simulink model "MG_2018b"  (R2020a)
settings: Solver=ode1  StartTime=0.0  StopTime=inf  FixedStep=2e-5  RelTol=1e-3  EnableMultiTasking=on
libraries: powerlib x26, powerlib_meascontrol x5, rtlab x3
settings Model: ARTEMISmethode_block_infos=$$__separator__$$  Creator=pengf  LastModifiedBy=mzh
settings SolverCC: AutoInsertRateTranBlk=on
settings DataIOCC: LimitDataPoints=on  SaveFormat=Array  SaveOutput=off  SaveTime=off  ReturnWorkspaceOutputs=off
settings OptimizationCC: LocalBlockOutputs=off  LifeSpan=inf
settings DebuggingCC: UnderspecifiedInitializationDetection=Classic  CheckExecutionContextPreStartOutputMsg=on  CheckExecutionContextRuntimeOutputMsg=on  SFUnexpectedBacktrackingDiag=warning  SFNoUnconditionalDefaultTransitionDiag=warning  SFExecutionAtInitializationDiag=none  ArithmeticOperatorsInVariantConditions=warning
settings HardwareCC: ProdBitPerPointer=32  ProdBitPerSizeT=32  ProdBitPerPtrDiffT=32  ProdLargestAtomicFloat=None  ProdIntDivRoundTo=Undefined  ProdEndianess=Unspecified  ProdWordSize=32  ProdHWDeviceType=32-bit Generic
settings ModelReferenceCC: PropagateSignalLabelsOutOfModel=off
settings SFSimCC: SimUseLocalCustomCode=off  CustomCodeUndefinedFunction=UseInterfaceOnly
settings RTWCC: RTWUseLocalCustomCode=off
settings CodeAppCC: StateflowObjectComments=on
settings GRTTargetCC: TargetLangStandard=C89/C90 (ANSI)  CombineOutputUpdateFcns=off  GRTInterface=on
settings ConfigComp: CovMetricSettings=dw  CovHtmlReporting=on  CovSaveCumulativeToWorkspaceVar=on  CovSaveSingleToWorkspaceVar=on  CovExternalEMLEnable=off
settings SimscapeCC: SimscapeNormalizeSystem=off

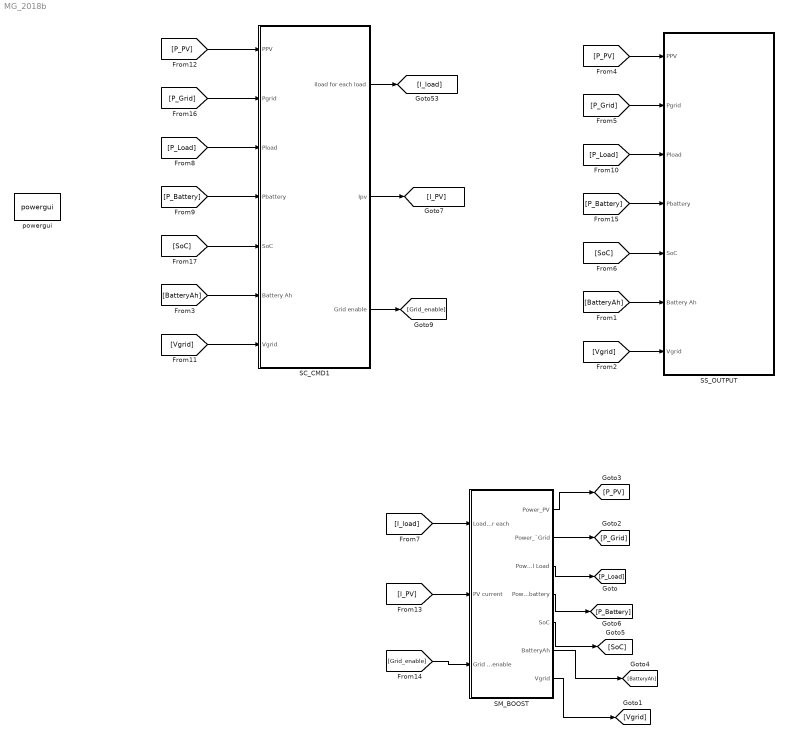
== system MG_2018b ==
  SC_CMD1 : Subsystem
  SM_BOOST : Subsystem
  SS_OUTPUT : Subsystem
  powergui : powerlib/powergui  Priority=1  SimulationMode=Discrete  SampleTime=2e-5  frequency=60  Iterations=50  frequencyindice=60  Pbase=100e6  ErrMax=1e-4  UnitsV=kV  UnitsW=MW  buscounter=0  FunctionMessages=off  echomessages=off  EnableUseOfTLC=off  CurrentSourceSwitches=off  DisableSnubberDevices=off  DisableRonSwitches=off  DisableVfSwitches=off  DisplayEquations=off  AutomaticDiscreteSolvers=off  SolverType=Tustin  Interpol=off  ExternalGateDelay=off  methode=off  Ts=100  x0status=blocks  SPID=off  SwTol=0  HookPort=off  NonlinearTolerance=1e-4  nMaxIteration=100  ContinueOnMaxIteration=off  RestoreLinks=warning  ResistiveCurrentMeasurement=off  Frange=[0:2:500]  Ylog=off  Xlog=on  ShowGrid=off  save=off  variable=ZData  structure=ScopeData3  ZoomFFT=off  StartTime=0.1  cycles=2  DisplayStyle=3  fundamental=50  FreqAxis=off  MaxFrequency=1000  frequencyindicesteady=1  RmsSteady=1  display=off
  wires:
  SC_CMD1/1(Iload for each load) -> [I_load]
  [P_PV] -> SC_CMD1/1(PPV)
  [P_Grid] -> SC_CMD1/2(Pgrid)
  [P_Grid] -> SS_OUTPUT/2(Pgrid)
  [I_load] -> SM_BOOST/1(Load current for each)
  [P_Battery] -> SC_CMD1/4(Pbattery)
  [SoC] -> SC_CMD1/5(SoC)
  [P_Battery] -> SS_OUTPUT/4(Pbattery)
  [Vgrid] -> SC_CMD1/7(Vgrid)
  [SoC] -> SS_OUTPUT/5(SoC)
  [P_Load] -> SC_CMD1/3("Pload ")
  [BatteryAh] -> SC_CMD1/6(Battery Ah)
  [P_PV] -> SS_OUTPUT/1(PPV)
  [P_Load] -> SS_OUTPUT/3("Pload ")
  SC_CMD1/2(Ipv) -> [I_PV]
  [I_PV] -> SM_BOOST/2(PV current)
  SM_BOOST/1(Power_PV) -> [P_PV]
  SM_BOOST/2(Power_`Grid) -> [P_Grid]
  SM_BOOST/3(Power_Total Load) -> [P_Load]
  SM_BOOST/4(Power_battery) -> [P_Battery]
  SM_BOOST/5(SoC) -> [SoC]
  SM_BOOST/6(BatteryAh) -> [BatteryAh]
  [Grid_enable] -> SM_BOOST/3(Grid connection enable)
  SM_BOOST/7("Vgrid ") -> [Vgrid]
  [BatteryAh] -> SS_OUTPUT/6(Battery Ah)
  [Vgrid] -> SS_OUTPUT/7(Vgrid)
  SC_CMD1/3(Grid enable) -> [Grid_enable]

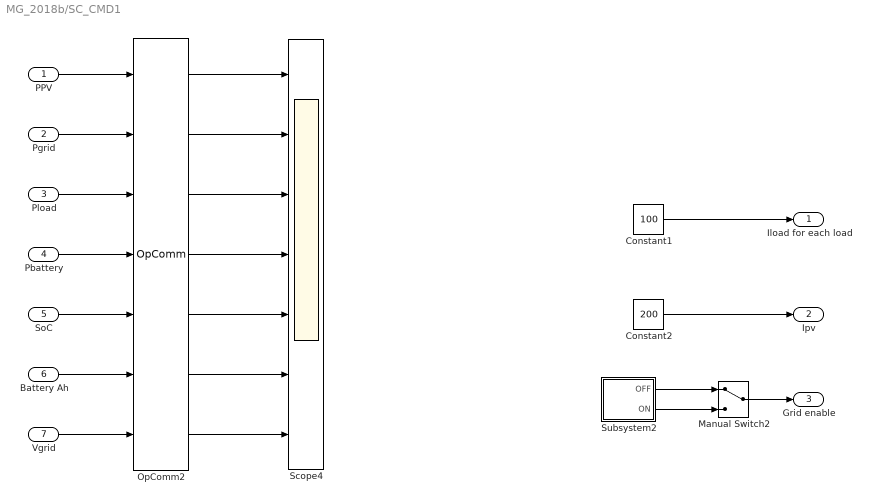
== system MG_2018b/SC_CMD1 ==
  PPV : Inport
  Pgrid : Inport  Port=2
  "Pload " : Inport  Port=3
  Pbattery : Inport  Port=4
  SoC : Inport  Port=5
  Battery Ah : Inport  Port=6
  Vgrid : Inport  Port=7
  Constant1 : Constant  Value=100
  Constant2 : Constant  Value=200
  Manual Switch2 : ManualSwitch
  OpComm2 : rtlab/OpComm  nbport=7  groupe_acq=1  subsys_rate=0  st=0  Synchronization=on  Interpolation=on  Threshold=1.0  Missed_Data=off  Sim_Time=off  Samples=off  dynSigOut=off  from_console=0  warning_done=off  writeOpCommFile=off  Offset=off
      settings: SourceProductName=RT-LAB
  Scope4 : Scope  NumInputPorts=7
  Subsystem2 : Subsystem
  Iload for each load : Outport
  Ipv : Outport  Port=2
  Grid enable : Outport  Port=3
  wires:
  Constant1/1 -> Iload for each load/1
  PPV/1 -> OpComm2/1
  Pgrid/1 -> OpComm2/2
  Pbattery/1 -> OpComm2/4
  SoC/1 -> OpComm2/5
  "Pload "/1 -> OpComm2/3
  Battery Ah/1 -> OpComm2/6
  Vgrid/1 -> OpComm2/7
  Constant2/1 -> Ipv/1
  OpComm2/1 -> Scope4/1
  OpComm2/2 -> Scope4/2
  OpComm2/3 -> Scope4/3
  OpComm2/4 -> Scope4/4
  OpComm2/5 -> Scope4/5
  OpComm2/6 -> Scope4/6
  OpComm2/7 -> Scope4/7
  Subsystem2/1(OFF) -> Manual Switch2/1
  Subsystem2/2(ON) -> Manual Switch2/2
  Manual Switch2/1 -> Grid enable/1

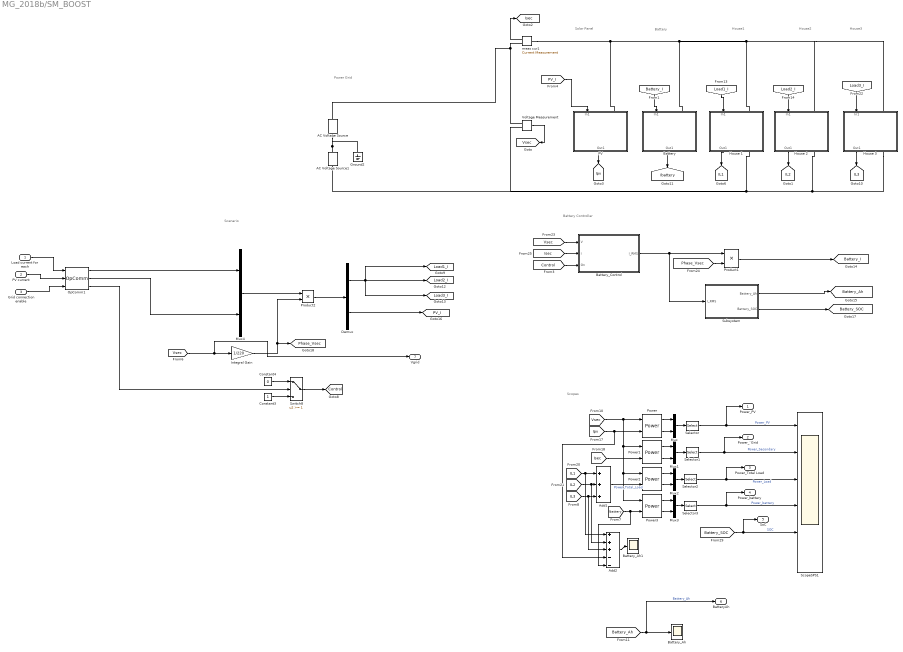
== system MG_2018b/SM_BOOST ==
  note: House1
  note: Solar Panel
  note: Scopes
  note: House3
  note: Battery Controller
  note: Battery
  note: House2
  note: Power Grid
  note: Scenario
  Load current for each : Inport
  PV current : Inport  Port=2
  Grid connection enable : Inport  Port=3
  AC Voltage Source : powerlib/Electrical Sources/AC Voltage Source  Amplitude=110  Phase=0  Frequency=60  SampleTime=0  Measurements=None  BusType=swing  Pref=10e3  Qref=0  Qmin=-inf  Qmax=+inf
  AC Voltage Source1 : powerlib/Electrical Sources/AC Voltage Source  Amplitude=110  Phase=0  Frequency=60  SampleTime=0  Measurements=None  BusType=swing  Pref=10e3  Qref=0  Qmin=-inf  Qmax=+inf
  Add1 : Sum  Inputs=+++
  Add2 : Sum  Inputs=+++--
  Battery : Subsystem
  Battery_Ah : Scope
  Battery_Ah1 : Scope
  Battery_Control : Subsystem
  Constant3 : Constant
  Constant4 : Constant  Value=0
  Demux : Demux  Outputs=2
  Ground2 : powerlib/Elements/Ground  LConnTagsString=a
  House 1 : Subsystem
  House 2 : Subsystem
  House 3 : Subsystem
  Integral Gain : Gain  Gain=1/220
  Mux{,1..4} (5 alike) : Mux  Inputs=2
  OpComm1 : rtlab/OpComm  nbport=3  groupe_acq=1  subsys_rate=0  st=0  Synchronization=on  Interpolation=on  Threshold=1.0  Missed_Data=off  Sim_Time=off  Samples=off  dynSigOut=off  from_console=1  warning_done=off  writeOpCommFile=off  Offset=off
      settings: SourceProductName=RT-LAB
  PV : Subsystem
  Power{,1..3} (4 alike) : powerlib_meascontrol/Measurements/Power  Freq=60  Vinit=[1, 0]  Iinit=[1, 0]  Ts=0
  Product1 : Product
  Product2 : Product
  ScopeSPS1 : Scope  NumInputPorts=6
  Selector{,1..3} (4 alike) : Selector  InputPortWidth=2  IndexOptions=Index vector (dialog)  Indices=1  OutputSizes=1
  Subsystem : Subsystem  mask{AH=100}
      mask prompts: AH "Capacity[Ah]"
  Switch8 : Switch  Threshold=1
  Voltage Measurement : powerlib/Measurements/Voltage Measurement  PhasorSimulation=off  OutputType=Complex  PSBequivalent=0
  meas cur1 : powerlib/Measurements/Current Measurement  PhasorSimulation=off  OutputType=Complex  PSBequivalent=0
  Power_PV : Outport
  Power_`Grid : Outport  Port=2
  Power_Total Load : Outport  Port=3
  Power_battery : Outport  Port=4
  SoC : Outport  Port=5
  BatteryAh : Outport  Port=6
  "Vgrid " : Outport  Port=7
  tag scope: Battery_Ah=global, Battery_I=global, Battery_SOC=global, Control=global, IL1=global, IL2=global, IL3=global, Ibattery=global, Ipv=global, Isec=global, Load1_I=global, Load2_I=global, Load3_I=global, PV_I=global, Phase_Vsec=global, Vsec=global
  wires:
  Load current for each/1 -> OpComm1/1
  PV current/1 -> OpComm1/2
  [Load3_I] -> House 3/1(In1)
  House 1/1(Out1) -> [IL1]
  [Vsec] -> Battery_Control/1(V)
  [Load1_I] -> House 1/1(In1)
  [PV_I] -> PV/1(In1)
  Subsystem/1(Battery_Ah) -> [Battery_Ah]
  Battery/1(Out1) -> [Ibattery]
  [Battery_I] -> Battery/1(In1)
  Subsystem/2(Battery_SOC) -> [Battery_SOC]
  meas cur1/1 -> [Isec]
  [Control] -> Battery_Control/3(On)
  Battery_Control/1(I_RMS) -> Subsystem/1(I_RMS), Product1/1
  PV/1(Out1) -> [Ipv]
  House 2/1(Out1) -> [IL2]
  House 3/1(Out1) -> [IL3]
  [Isec] -> Battery_Control/2(I)
  [Phase_Vsec] -> Product1/2
  [Load2_I] -> House 2/1(In1)
  Voltage Measurement/1 -> [Vsec]
  Selector/1 -> Power_PV/1, ScopeSPS1/1  "Power_PV"
  [Vsec] -> Power1/1, Power3/1, Power2/1, Power/1
  Add1/1 -> Power2/2  "Power_Total_Load"
  [Isec] -> Power1/2
  [Ipv] -> Add2/4, Power/2
  Selector3/1 -> Power_battery/1, ScopeSPS1/4  "Power_battery"
  [Battery_SOC] -> SoC/1, ScopeSPS1/5  "SOC"
  [IL3] -> Add2/3, Add1/3
  Power/1 -> Mux/1
  [IL1] -> Add2/1, Add1/1
  [Battery_Ah] -> BatteryAh/1, Battery_Ah/1  "Battery_Ah"
  Power/2 -> Mux/2
  Selector2/1 -> Power_Total Load/1, ScopeSPS1/3  "Power_Load"
  Power1/1 -> Mux1/1
  Power3/2 -> Mux3/2
  Power2/1 -> Mux2/1
  Selector1/1 -> Power_`Grid/1, ScopeSPS1/2  "Power_Secondary"
  Power1/2 -> Mux1/2
  Power3/1 -> Mux3/1
  Mux3/1 -> Selector3/1
  Mux2/1 -> Selector2/1
  Mux/1 -> Selector/1
  Mux1/1 -> Selector1/1
  Add2/1 -> Battery_Ah1/1
  Power2/2 -> Mux2/2
  [Ibattery] -> Add2/5, Power3/2
  [IL2] -> Add2/2, Add1/2
  Mux4/1 -> Product2/1
  Integral Gain/1 -> [Phase_Vsec], Product2/2
  OpComm1/3 -> Switch8/2
  OpComm1/2 -> Mux4/2
  OpComm1/1 -> Mux4/1
  [Vsec] -> "Vgrid "/1, Integral Gain/1
  Constant3/1 -> Switch8/3
  Product2/1 -> Demux/1
  Constant4/1 -> Switch8/1
  Switch8/1 -> [Control]
  Grid connection enable/1 -> OpComm1/3
  Product1/1 -> [Battery_I]
  Demux/1 -> [Load3_I], [Load2_I], [Load1_I]
  Demux/2 -> [PV_I]
  connections:
  AC Voltage Source1/RConn1 -- AC Voltage Source/LConn1 -- Ground2/LConn1
  Voltage Measurement/LConn1 -- AC Voltage Source/RConn1 -- meas cur1/RConn1
  House 2/RConn1 -- House 3/RConn1 -- AC Voltage Source1/LConn1 -- Voltage Measurement/LConn2 -- House 1/RConn1
  Battery/LConn1 -- House 3/LConn1 -- House 2/LConn1 -- House 1/LConn1 -- meas cur1/LConn1 -- PV/LConn1

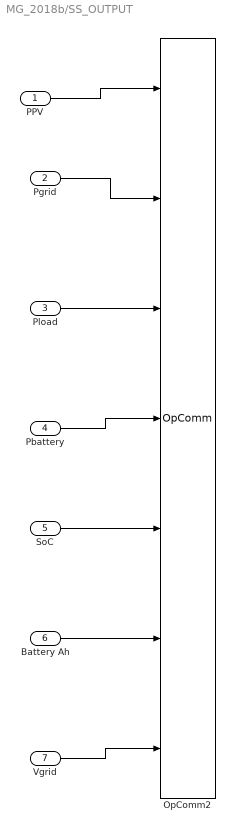
== system MG_2018b/SS_OUTPUT ==
  PPV : Inport
  Pgrid : Inport  Port=2
  "Pload " : Inport  Port=3
  Pbattery : Inport  Port=4
  SoC : Inport  Port=5
  Battery Ah : Inport  Port=6
  Vgrid : Inport  Port=7
  OpComm2 : rtlab/OpComm  nbport=7  groupe_acq=1  subsys_rate=0  st=0  Synchronization=on  Interpolation=on  Threshold=1.0  Missed_Data=off  Sim_Time=off  Samples=off  dynSigOut=off  from_console=0  warning_done=off  writeOpCommFile=off  Offset=off
      settings: SourceProductName=RT-LAB
  wires:
  Pgrid/1 -> OpComm2/2
  PPV/1 -> OpComm2/1
  "Pload "/1 -> OpComm2/3
  Pbattery/1 -> OpComm2/4
  SoC/1 -> OpComm2/5
  Battery Ah/1 -> OpComm2/6
  Vgrid/1 -> OpComm2/7

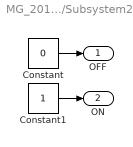
== system MG_2018b/SC_CMD1/Subsystem2 ==
  Constant : Constant  Value=0
  Constant1 : Constant
  OFF : Outport
  ON : Outport  Port=2
  wires:
  Constant/1 -> OFF/1
  Constant1/1 -> ON/1

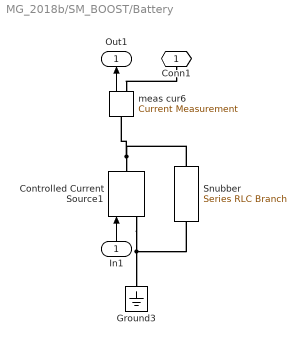
== system MG_2018b/SM_BOOST/Battery ==
  In1 : Inport
  Controlled Current Source1 : powerlib/Electrical Sources/Controlled Current Source  Initialize=on  Source_Type=AC  Amplitude=0  Phase=30  Frequency=60  Measurements=None
  Ground3 : powerlib/Elements/Ground  LConnTagsString=a
  Snubber : powerlib/Elements/Series RLC Branch  LConnTagsString=__new0  RConnTagsString=__new0  BranchType=R  Resistance=1e6  Inductance=1e-3  SetiL0=off  InitialCurrent=0  Capacitance=1e-6  Setx0=off  InitialVoltage=0  Measurements=None
  meas cur6 : powerlib/Measurements/Current Measurement  PhasorSimulation=off  OutputType=Complex  PSBequivalent=0
  Conn1 : PMIOPort  Side=Left
  Out1 : Outport  VectorParamsAs1DForOutWhenUnconnected=off
  wires:
  meas cur6/1 -> Out1/1
  In1/1 -> Controlled Current Source1/1
  connections:
  Controlled Current Source1/LConn1 -- Ground3/LConn1 -- Snubber/RConn1
  Controlled Current Source1/RConn1 -- Snubber/LConn1 -- meas cur6/LConn1
  Conn1/RConn1 -- meas cur6/RConn1

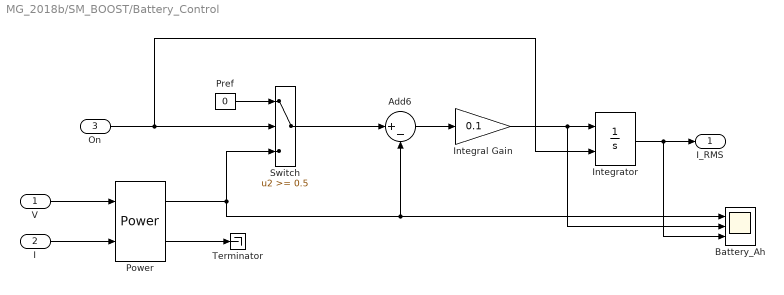
== system MG_2018b/SM_BOOST/Battery_Control ==
  V : Inport
  I : Inport  Port=2
  On : Inport  Port=3
  Add6 : Sum  Inputs=|+-
  Battery_Ah : Scope  NumInputPorts=3
  Integral Gain : Gain  Gain=0.1
  Integrator : Integrator  ExternalReset=falling  LimitOutput=on  UpperSaturationLimit=500  LowerSaturationLimit=-500
  Power : powerlib_meascontrol/Measurements/Power  Freq=60  Vinit=[1, 0]  Iinit=[1, 0]  Ts=0
  Pref : Constant  Value=0
  Switch : Switch  Threshold=0.5
  Terminator : Terminator
  I_RMS : Outport  OutputWhenDisabled=reset  InitialOutput=0  VectorParamsAs1DForOutWhenUnconnected=off
  wires:
  Pref/1 -> Switch/1
  Integrator/1 -> Battery_Ah/3, I_RMS/1
  On/1 -> Integrator/2, Switch/2
  Add6/1 -> Integral Gain/1
  Integral Gain/1 -> Battery_Ah/2, Integrator/1
  Power/1 -> Switch/3, Add6/2, Battery_Ah/1
  I/1 -> Power/2
  V/1 -> Power/1
  Power/2 -> Terminator/1
  Switch/1 -> Add6/1

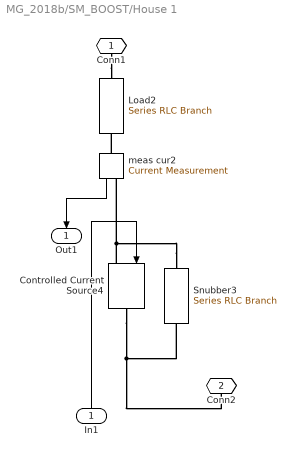
== system MG_2018b/SM_BOOST/House 1 ==
  In1 : Inport
  Controlled Current Source4 : powerlib/Electrical Sources/Controlled Current Source  Initialize=on  Source_Type=AC  Amplitude=0  Phase=30  Frequency=60  Measurements=None
  Load2 : powerlib/Elements/Series RLC Branch  LConnTagsString=__new0  RConnTagsString=__new0  BranchType=R  Resistance=16  Inductance=1e-3  SetiL0=off  InitialCurrent=0  Capacitance=1e-6  Setx0=off  InitialVoltage=0  Measurements=None
  Snubber3 : powerlib/Elements/Series RLC Branch  LConnTagsString=__new0  RConnTagsString=__new0  BranchType=R  Resistance=1e6  Inductance=1e-3  SetiL0=off  InitialCurrent=0  Capacitance=1e-6  Setx0=off  InitialVoltage=0  Measurements=None
  meas cur2 : powerlib/Measurements/Current Measurement  PhasorSimulation=off  OutputType=Complex  PSBequivalent=0
  Conn1 : PMIOPort  Side=Left
  Conn2 : PMIOPort  Port=2  Side=Right
  Out1 : Outport  VectorParamsAs1DForOutWhenUnconnected=off
  wires:
  In1/1 -> Controlled Current Source4/1
  meas cur2/1 -> Out1/1
  connections:
  Conn1/RConn1 -- Load2/LConn1
  meas cur2/LConn1 -- Load2/RConn1
  Snubber3/LConn1 -- Controlled Current Source4/LConn1 -- meas cur2/RConn1
  Snubber3/RConn1 -- Controlled Current Source4/RConn1 -- Conn2/RConn1

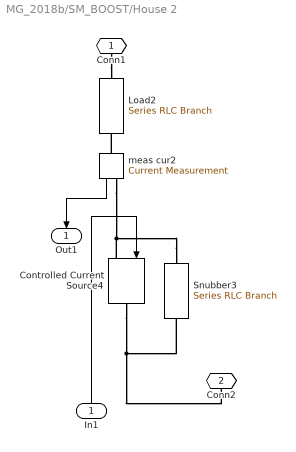
== system MG_2018b/SM_BOOST/House 2 ==
  In1 : Inport
  Controlled Current Source4 : powerlib/Electrical Sources/Controlled Current Source  Initialize=on  Source_Type=AC  Amplitude=0  Phase=30  Frequency=60  Measurements=None
  Load2 : powerlib/Elements/Series RLC Branch  LConnTagsString=__new0  RConnTagsString=__new0  BranchType=R  Resistance=16  Inductance=1e-3  SetiL0=off  InitialCurrent=0  Capacitance=1e-6  Setx0=off  InitialVoltage=0  Measurements=None
  Snubber3 : powerlib/Elements/Series RLC Branch  LConnTagsString=__new0  RConnTagsString=__new0  BranchType=R  Resistance=1e6  Inductance=1e-3  SetiL0=off  InitialCurrent=0  Capacitance=1e-6  Setx0=off  InitialVoltage=0  Measurements=None
  meas cur2 : powerlib/Measurements/Current Measurement  PhasorSimulation=off  OutputType=Complex  PSBequivalent=0
  Conn1 : PMIOPort  Side=Left
  Conn2 : PMIOPort  Port=2  Side=Right
  Out1 : Outport  VectorParamsAs1DForOutWhenUnconnected=off
  wires:
  meas cur2/1 -> Out1/1
  In1/1 -> Controlled Current Source4/1
  connections:
  meas cur2/LConn1 -- Load2/RConn1
  Conn1/RConn1 -- Load2/LConn1
  Snubber3/LConn1 -- meas cur2/RConn1 -- Controlled Current Source4/LConn1
  Conn2/RConn1 -- Controlled Current Source4/RConn1 -- Snubber3/RConn1

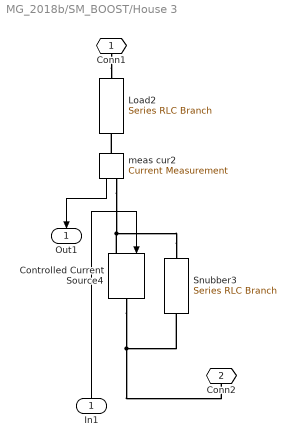
== system MG_2018b/SM_BOOST/House 3 ==
  In1 : Inport
  Controlled Current Source4 : powerlib/Electrical Sources/Controlled Current Source  Initialize=on  Source_Type=AC  Amplitude=0  Phase=30  Frequency=60  Measurements=None
  Load2 : powerlib/Elements/Series RLC Branch  LConnTagsString=__new0  RConnTagsString=__new0  BranchType=R  Resistance=16  Inductance=1e-3  SetiL0=off  InitialCurrent=0  Capacitance=1e-6  Setx0=off  InitialVoltage=0  Measurements=None
  Snubber3 : powerlib/Elements/Series RLC Branch  LConnTagsString=__new0  RConnTagsString=__new0  BranchType=R  Resistance=1e6  Inductance=1e-3  SetiL0=off  InitialCurrent=0  Capacitance=1e-6  Setx0=off  InitialVoltage=0  Measurements=None
  meas cur2 : powerlib/Measurements/Current Measurement  PhasorSimulation=off  OutputType=Complex  PSBequivalent=0
  Conn1 : PMIOPort  Side=Left
  Conn2 : PMIOPort  Port=2  Side=Right
  Out1 : Outport  VectorParamsAs1DForOutWhenUnconnected=off
  wires:
  meas cur2/1 -> Out1/1
  In1/1 -> Controlled Current Source4/1
  connections:
  Conn1/RConn1 -- Load2/LConn1
  meas cur2/LConn1 -- Load2/RConn1
  Snubber3/LConn1 -- meas cur2/RConn1 -- Controlled Current Source4/LConn1
  Conn2/RConn1 -- Controlled Current Source4/RConn1 -- Snubber3/RConn1

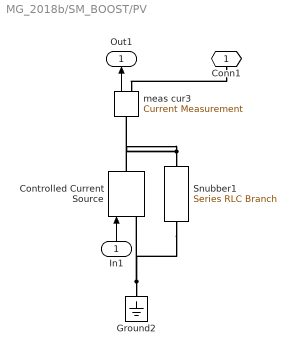
== system MG_2018b/SM_BOOST/PV ==
  In1 : Inport
  Controlled Current Source : powerlib/Electrical Sources/Controlled Current Source  Initialize=on  Source_Type=AC  Amplitude=0  Phase=30  Frequency=60  Measurements=None
  Ground2 : powerlib/Elements/Ground  LConnTagsString=a
  Snubber1 : powerlib/Elements/Series RLC Branch  LConnTagsString=__new0  RConnTagsString=__new0  BranchType=R  Resistance=1e6  Inductance=1e-3  SetiL0=off  InitialCurrent=0  Capacitance=1e-6  Setx0=off  InitialVoltage=0  Measurements=None
  meas cur3 : powerlib/Measurements/Current Measurement  PhasorSimulation=off  OutputType=Complex  PSBequivalent=0
  Conn1 : PMIOPort  Side=Left
  Out1 : Outport  VectorParamsAs1DForOutWhenUnconnected=off
  wires:
  meas cur3/1 -> Out1/1
  In1/1 -> Controlled Current Source/1
  connections:
  Ground2/LConn1 -- Controlled Current Source/LConn1 -- Snubber1/RConn1
  Snubber1/LConn1 -- Controlled Current Source/RConn1 -- meas cur3/LConn1
  Conn1/RConn1 -- meas cur3/RConn1

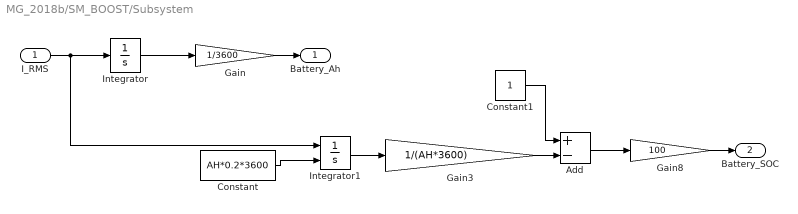
== system MG_2018b/SM_BOOST/Subsystem ==
  I_RMS : Inport
  Add : Sum  Inputs=+-
  Constant : Constant  Value=AH*0.2*3600
  Constant1 : Constant
  Gain : Gain  Gain=1/3600
  Gain3 : Gain  Gain=1/(AH*3600)
  Gain8 : Gain  Gain=100
  Integrator : Integrator
  Integrator1 : Integrator  InitialConditionSource=external
  Battery_Ah : Outport  VectorParamsAs1DForOutWhenUnconnected=off
  Battery_SOC : Outport  Port=2  VectorParamsAs1DForOutWhenUnconnected=off
  wires:
  Integrator/1 -> Gain/1
  Integrator1/1 -> Gain3/1
  Gain3/1 -> Add/2
  Constant1/1 -> Add/1
  Add/1 -> Gain8/1
  Constant/1 -> Integrator1/2
  I_RMS/1 -> Integrator/1, Integrator1/1
  Gain/1 -> Battery_Ah/1
  Gain8/1 -> Battery_SOC/1
